simulink model "Freqeunzbereichregler_Simulation"  (R2021b)
settings: Solver=ode23  StartTime=0.0  StopTime=5000  RelTol=1e-3
settings Model: Creator=liams  LastModifiedBy=liams

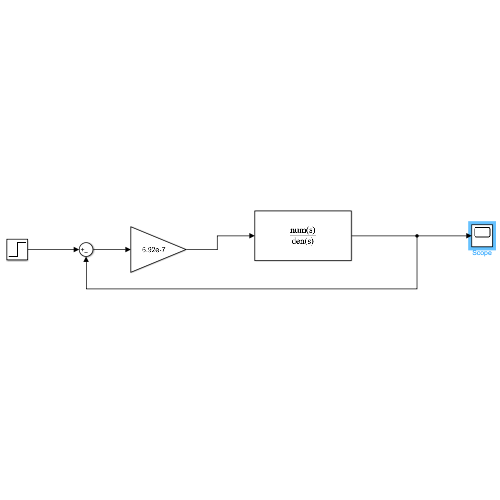
[thumbnail: Simulink's stored preview of the top-level diagram]
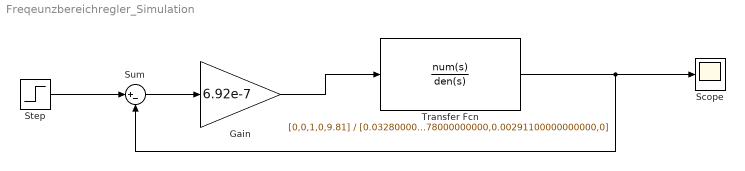
== system Freqeunzbereichregler_Simulation ==
  Gain : Gain  Gain=6.92e-7
  Scope : Scope
  Step : Step  SampleTime=0
  Sum : Sum  Inputs=|+-
  Transfer Fcn : TransferFcn  Numerator=[0,0,1,0,9.81]  Denominator=[0.0328000000000000,0.000295200000000000,0.723978000000000,0.00291100000000000,0]
  wires:
  Gain/1 -> Transfer Fcn/1
  Step/1 -> Sum/1
  Sum/1 -> Gain/1
  Transfer Fcn/1 -> Sum/2, Scope/1
